simulink model "ITCG_2D_simulation"  (R2023b)
settings: Solver=FixedStepAuto  StartTime=0.0  StopTime=45  FixedStep=1/100  RelTol=1e-3
values from neighbouring files (symbols this model uses):
  k = g    [ITCG_sim.m]    (also in data_analysis.m = 1.5)
  M = j    [ITCG_sim.m]    (also in data_analysis.m = 10)
  N = i    [ITCG_sim.m]    (also in data_analysis.m = 3)
  t_d = l    [ITCG_sim.m]    (also in data_analysis.m = td_range(i))
libraries: simulink x1
settings Model: Creator=Administrator  LastModifiedBy=Administrator
settings DebuggingCC: UnderSpecifiedDimensionMsg=warning

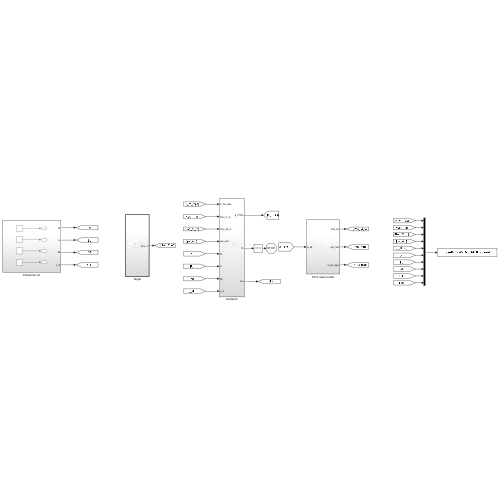
[thumbnail: Simulink's stored preview of the top-level diagram]
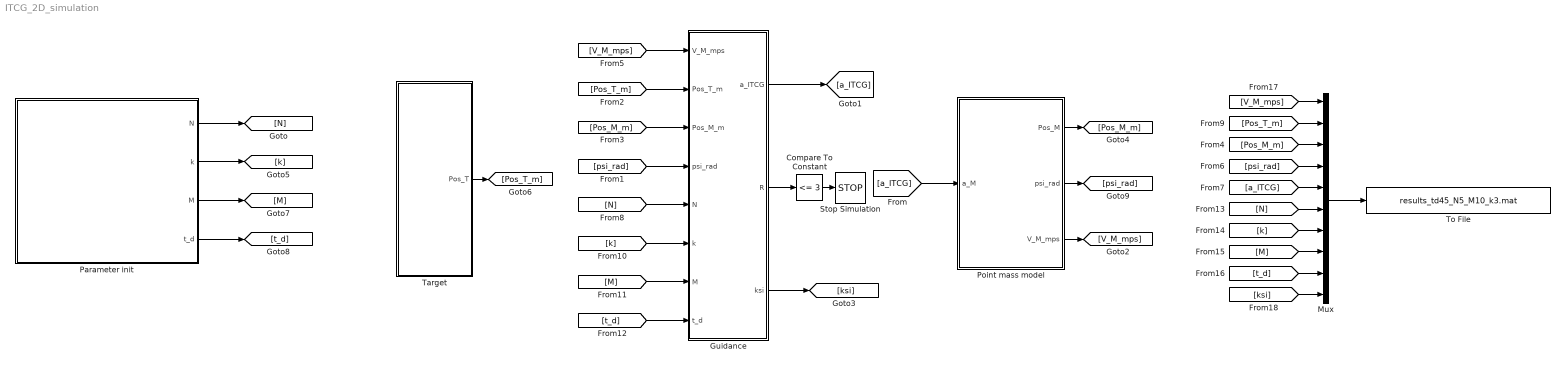
== system ITCG_2D_simulation ==
  Compare To Constant : simulink/Logic and Bit Operations/Compare To Constant  relop=<=  const=3  OutDataTypeStr=boolean
  Guidance : Subsystem
  Mux : Mux  Inputs=10
  Parameter init : Subsystem
  Point mass model : Subsystem
  Stop Simulation : Stop
  Target : Subsystem  TreatAsAtomicUnit=on
  To File : ToFile  Filename=results_td45_N5_M10_k3.mat
  wires:
  [Pos_M_m] -> Guidance/3(Pos_M_m)
  [psi_rad] -> Guidance/4(psi_rad)
  [Pos_T_m] -> Guidance/2(Pos_T_m)
  Target/1(Pos_T) -> [Pos_T_m]
  Point mass model/2(psi_rad) -> [psi_rad]
  [V_M_mps] -> Guidance/1(V_M_mps)
  Point mass model/3(V_M_mps) -> [V_M_mps]
  [a_ITCG] -> Point mass model/1(a_M)
  Point mass model/1(Pos_M) -> [Pos_M_m]
  [N] -> Guidance/5(N)
  [k] -> Guidance/6(k)
  [M] -> Guidance/7(M)
  [t_d] -> Guidance/8(t_d)
  Parameter init/1(N) -> [N]
  Parameter init/2(k) -> [k]
  Parameter init/3(M) -> [M]
  Parameter init/4(t_d) -> [t_d]
  [V_M_mps] -> Mux/1
  [Pos_T_m] -> Mux/2
  [Pos_M_m] -> Mux/3
  [psi_rad] -> Mux/4
  [a_ITCG] -> Mux/5
  [N] -> Mux/6
  [k] -> Mux/7
  [M] -> Mux/8
  [t_d] -> Mux/9
  Mux/1 -> To File/1
  Guidance/2(R) -> Compare To Constant/1
  Compare To Constant/1 -> Stop Simulation/1
  Guidance/1(a_ITCG) -> [a_ITCG]
  Guidance/3(ksi) -> [ksi]
  [ksi] -> Mux/10

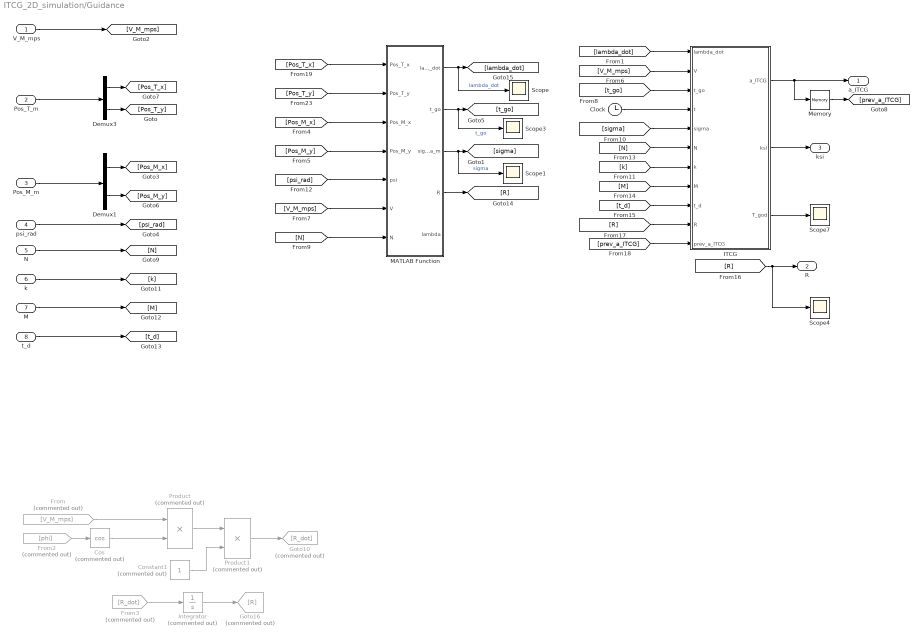
== system ITCG_2D_simulation/Guidance ==
  V_M_mps : Inport
  Pos_T_m : Inport  Port=2
  Pos_M_m : Inport  Port=3
  psi_rad : Inport  Port=4
  N : Inport  Port=5
  k : Inport  Port=6
  M : Inport  Port=7
  t_d : Inport  Port=8
  Clock : Clock
  Constant1 : Constant  Commented=on
  Cos : Trigonometry  Commented=on  Operator=cos
  Demux1 : Demux  Outputs=2
  Demux3 : Demux  Outputs=2
  From : From  Commented=on  GotoTag=V_M_mps
  From2 : From  Commented=on  GotoTag=phi
  From3 : From  Commented=on  GotoTag=R_dot
  Goto10 : Goto  Commented=on  GotoTag=R_dot
  Goto16 : Goto  Commented=on  GotoTag=R
  ITCG : MATLAB Function  TreatAsAtomicUnit=on
  Integrator : Integrator  Commented=on
  MATLAB Function : MATLAB Function  TreatAsAtomicUnit=on
  Memory : Memory
  Product : Product  Commented=on
  Product1 : Product  Commented=on
  Scope{,1,3..4,7} (5 alike) : Scope
  a_ITCG : Outport
  R : Outport  Port=2
  ksi : Outport  Port=3
  wires:
  ITCG/1(a_ITCG) -> Memory/1, a_ITCG/1
  V_M_mps/1 -> [V_M_mps]
  [V_M_mps] -> ITCG/2(V)
  [lambda_dot] -> ITCG/1(lambda_dot)
  [V_M_mps] -> MATLAB Function/6(V)
  psi_rad/1 -> [psi_rad]
  Pos_T_m/1 -> Demux3/1
  Demux3/1 -> [Pos_T_x]
  Demux1/2 -> [Pos_M_y]
  Pos_M_m/1 -> Demux1/1
  Demux1/1 -> [Pos_M_x]
  Demux3/2 -> [Pos_T_y]
  MATLAB Function/1(lambda_dot) -> Scope/1, [lambda_dot]  "lambda_dot"
  MATLAB Function/2(t_go) -> Scope3/1, [t_go]  "t_go"
  Clock/1 -> ITCG/4(t)
  From2/1 -> Cos/1
  From/1 -> Product/1
  Cos/1 -> Product/2
  Product/1 -> Product1/1
  Constant1/1 -> Product1/2
  Product1/1 -> Goto10/1
  From3/1 -> Integrator/1
  Integrator/1 -> Goto16/1
  [Pos_M_x] -> MATLAB Function/3(Pos_M_x)
  [Pos_M_y] -> MATLAB Function/4(Pos_M_y)
  [Pos_T_x] -> MATLAB Function/1(Pos_T_x)
  [Pos_T_y] -> MATLAB Function/2(Pos_T_y)
  [psi_rad] -> MATLAB Function/5(psi)
  MATLAB Function/3(sigma_m) -> Scope1/1, [sigma]  "sigma"
  [t_go] -> ITCG/3(t_go)
  [sigma] -> ITCG/5(sigma)
  ITCG/2(ksi) -> ksi/1
  N/1 -> [N]
  t_d/1 -> [t_d]
  M/1 -> [M]
  k/1 -> [k]
  [N] -> MATLAB Function/7(N)
  [N] -> ITCG/6(N)
  [k] -> ITCG/7(k)
  [M] -> ITCG/8(M)
  [t_d] -> ITCG/9(t_d)
  MATLAB Function/4(R) -> [R]
  [R] -> Scope4/1, R/1
  [R] -> ITCG/10(R)
  Memory/1 -> [prev_a_ITCG]
  [prev_a_ITCG] -> ITCG/11(prev_a_ITCG)
  ITCG/3(T_god) -> Scope7/1

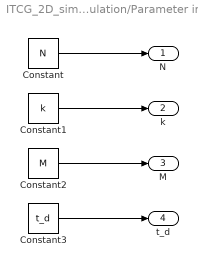
== system ITCG_2D_simulation/Parameter init ==
  Constant : Constant  Value=N
  Constant1 : Constant  Value=k
  Constant2 : Constant  Value=M
  Constant3 : Constant  Value=t_d
  N : Outport
  k : Outport  Port=2
  M : Outport  Port=3
  t_d : Outport  Port=4
  wires:
  Constant/1 -> N/1
  Constant1/1 -> k/1
  Constant2/1 -> M/1
  Constant3/1 -> t_d/1

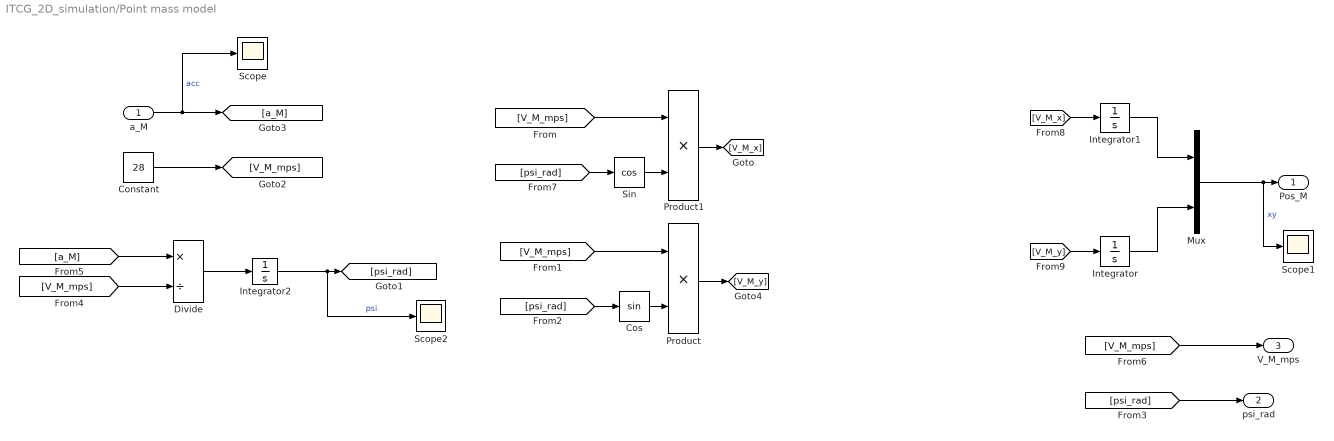
== system ITCG_2D_simulation/Point mass model ==
  a_M : Inport
  Constant : Constant  Value=28
  Cos : Trigonometry
  Divide : Product  Inputs=*/
  Integrator : Integrator
  Integrator1 : Integrator
  Integrator2 : Integrator  InitialCondition=90*pi/180
  Mux : Mux  Inputs=2
  Product : Product
  Product1 : Product
  Scope : Scope
  Scope1 : Scope
  Scope2 : Scope
  Sin : Trigonometry  Operator=cos
  Pos_M : Outport
  psi_rad : Outport  Port=2
  V_M_mps : Outport  Port=3
  wires:
  [V_M_mps] -> Product1/1
  [V_M_mps] -> Product/1
  [psi_rad] -> Sin/1
  [psi_rad] -> Cos/1
  Cos/1 -> Product/2
  Sin/1 -> Product1/2
  Mux/1 -> Scope1/1, Pos_M/1  "xy"
  [psi_rad] -> psi_rad/1
  Integrator/1 -> Mux/2
  Integrator1/1 -> Mux/1
  Divide/1 -> Integrator2/1
  [V_M_mps] -> Divide/2
  Constant/1 -> [V_M_mps]
  [V_M_mps] -> V_M_mps/1
  [a_M] -> Divide/1
  a_M/1 -> Scope/1, [a_M]  "acc"
  Product1/1 -> [V_M_x]
  Product/1 -> [V_M_y]
  [V_M_x] -> Integrator1/1
  [V_M_y] -> Integrator/1
  Integrator2/1 -> Scope2/1, [psi_rad]  "psi"

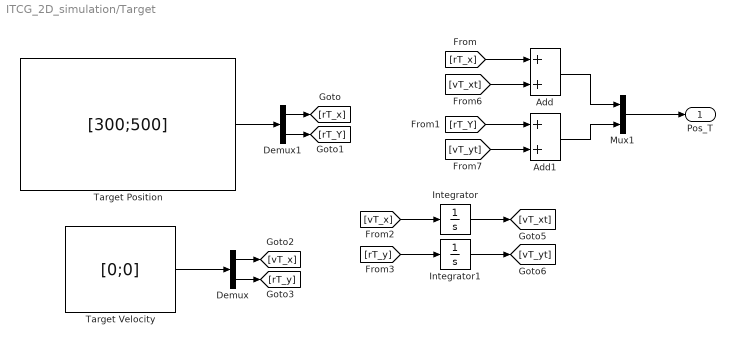
== system ITCG_2D_simulation/Target ==
  Add : Sum
  Add1 : Sum
  Demux : Demux  Outputs=2
  Demux1 : Demux  Outputs=2
  Integrator : Integrator
  Integrator1 : Integrator
  Mux1 : Mux  Inputs=2
  Target Position : Constant  Value=[300;500]  VectorParams1D=off
  Target Velocity : Constant  Value=[0;0]  VectorParams1D=off
  Pos_T : Outport
  wires:
  Target Velocity/1 -> Demux/1
  Target Position/1 -> Demux1/1
  Add/1 -> Mux1/1
  Add1/1 -> Mux1/2
  Mux1/1 -> Pos_T/1
  Demux1/1 -> [rT_x]
  [rT_x] -> Add/1
  Demux1/2 -> [rT_Y]
  [rT_Y] -> Add1/1
  Demux/1 -> [vT_x]
  Demux/2 -> [rT_y]
  [vT_xt] -> Add/2
  [vT_yt] -> Add1/2
  [vT_x] -> Integrator/1
  [rT_y] -> Integrator1/1
  Integrator/1 -> [vT_xt]
  Integrator1/1 -> [vT_yt]

== matlab function ITCG_2D_simulation/Guidance/MATLAB Function ==
  data: Pos_T_x input; lambda_dot output; Pos_T_y input; Pos_M_x input; Pos_M_y input; psi input; V input; N input; t_go output; sigma_m output; R output; lambda output
function [lambda_dot, t_go, sigma_m, R, lambda] = fcn(Pos_T_x, Pos_T_y, Pos_M_x, Pos_M_y, psi, V, N)
    R2D=180/pi;
    D2R=pi/180;
    % relative parameter
    rTM_x = Pos_T_x - Pos_M_x;
    rTM_y = Pos_T_y - Pos_M_y;
    R=sqrt((rTM_x)^2+(rTM_y)^2);    
    lambda=atan2(rTM_y,rTM_x); % atan2를 사용하여 0 처리 및 사분면 처리
    sigma=psi-lambda;
    sigma_m=abs(mod(sigma+pi, 2*pi)-pi);
    % R_dot=-V*cos(phi);

    % a=1/(2*(N-1));
    % b=1/2;
    % 
    % B1 = integral(@(t) t.^(a-1) .* (1-t).^(b-1), 0, sin(sigma_m)^2, "AbsTol", 1e-10, "RelTol", 1e-4);
    % B2 = beta(a, b);
    % 
    % if isnan(B1)
    %     B1 = 0;
    % end
    % if isnan(B2)
    %     B2 = 0;
    % end
    % 
    % if sigma_m >= 0 && sigma_m < pi/2
    %     t_go = (R / (2*V*(N-1)*sin(sigma_m)^(1/(N-1)))) * B1;
    %     if isinf(t_go) || t_go <= 0.1
    %         t_go = 1e-3;
    %     end
    % elseif sigma_m >= pi/2 && sigma_m <= pi
    %     t_go = (R / (2*V*(N-1)*sin(sigma_m)^(1/(N-1)))) * (2*B2 - B1);
    %     if isinf(t_go) || t_go <= 0.1
    %         t_go = 1e-3;
    %     end
    % else
    %     t_go = 0;
    % end
    
    t_go = R/V*(1+(sigma_m^2/(2*(2*N-1))));

    % PNG command
    lambda_dot = -V*sin(sigma_m)/R;

    % if R<10
    %     lambda_dot=0;
    % end
end

== matlab function ITCG_2D_simulation/Guidance/ITCG ==
  data: a_ITCG output; lambda_dot input; V input; t_go input; t input; sigma input; ksi output; N input; k input; M input; t_d input; T_god output; R input; prev_a_ITCG input
function [a_ITCG, ksi, T_god]  = fcn(lambda_dot, V, t_go, t, sigma, N, k, M, t_d, R, prev_a_ITCG)


T_god=t_d-t;
ksi=t_go-T_god;
% if ksi>-1e-1
%     ksi=0;
% end
sgmf_ksi = 2*( (1/(1+exp(-10*ksi))) - 1/2);
% sgmf_abs_sigma = 2*( 1/(1+exp(-abs(sigma))) - 1/2);
%
%ITCG command
% a_ITCG = N*(1+k*sign(ksi))*V*theta_dot + M*(sign(abs(phi))-1)*sign(ksi);

if R <10
    a_ITCG = prev_a_ITCG;
else
    a_ITCG = N*(1+k*sgmf_ksi)*V*lambda_dot;
end



% a_ITCG = N*(1+k*sgmf_ksi)*V*lambda_dot + M*(sgmf_abs_sigma-1)*sgmf_ksi;
% function [a_ITCG, ksi, T_god]  = fcn(lambda_dot, V, t_go, t, sigma, N, k, M, t_d, R, prev_a_ITCG)
% 
% T_god = t_d-t;
% ksi = t_go-T_god;
% 
% sigma_deg = sigma * 180/pi;
% 
% sgmf_ksi = 2*( 1/(1+exp(-10*ksi)) - 1/2);
% sgmf_abs_sigma = 2*( 1/(1+exp(-10*abs(sigma_deg))) - 1/2);
% 
% a_ITCG = N*(1+k*sgmf_ksi)*V*lambda_dot + M*(sgmf_abs_sigma-1)*sgmf_ksi*0;
% 
% term = M*(sgmf_abs_sigma-1)*sgmf_ksi;
% 
% if R <10
%     a_ITCG = prev_a_ITCG;
% else
%     a_ITCG = N*(1+k*sgmf_ksi)*V*lambda_dot;
% end
